simulink model "VisionModel_v16_3"  (Simulink 7.6)
settings: Solver=FixedStepDiscrete  StartTime=0.0  StopTime=0  RelTol=1e-3
undefined symbols (not defined in the file or in its folder): Rec, SDTV
libraries: vipconversions x4, vipgeotforms x3
settings Model: Creator=Administrator  LastModifiedBy=root
settings OptimizationCC: OptimizeModelRefInitCode=on
settings RTWCC: SystemTargetFile=ert.tlc  GenCodeOnly=on  TemplateMakefile=ert_default_tmf  PostCodeGenCommand=packNGo(buildInfo, {'packType' 'flat'})  Description=Real-Time Workshop Embedded Coder  GenerateReport=on  ProcessScript=ert_make_rtw_hook  IncludeHyperlinkInReport=on  LaunchReport=on  TargetLang=C++
settings CodeAppCC: IgnoreCustomStorageClasses=off
settings ERTTargetCC: MultiwordLength=2048  GenerateSampleERTMain=on  IncludeMdlTerminateFcn=off  ERTCustomFileTemplate=example_file_process.tlc  ConvertIfToSwitch=off

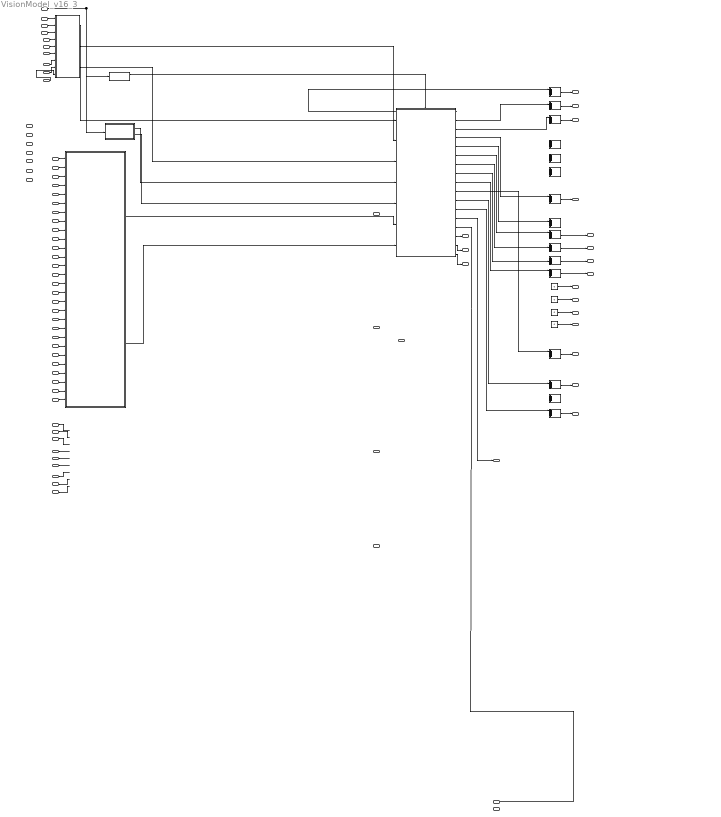
== system VisionModel_v16_3 ==
  note: Forward camera QImage array
  note: Down camera QImage array
  note: Forward
  note: Down
  note: Current target information
  note: Desired target information
  note: Mode and general target information
  note: Note: TargetFound, and the last three inputs to MotionController.mdl,
      | can be changed by the script, not the vision model.
  note: Path-following variables
      | DesiredPathDirection:
      | 0 = Use internal default
      | 1 = Take left path
      | 2 = Take right path
  R_forward_in : Inport  PortDimensions=Forward_Camera_Dimensions
  G_forward_in : Inport  Port=2  PortDimensions=Forward_Camera_Dimensions
  B_forward_in : Inport  Port=3  PortDimensions=Forward_Camera_Dimensions
  R_down_in : Inport  Port=4  PortDimensions=Down_Camera_Dimensions
  G_down_in : Inport  Port=5  PortDimensions=Down_Camera_Dimensions
  B_down_in : Inport  Port=6  PortDimensions=Down_Camera_Dimensions
  ModeSelect : Inport  Port=7
  OutputImage : Inport  Port=8
  DesiredPathDirection : Inport  Port=9
  DesiredBuoyColor : Inport  Port=10
  DesiredTorpedoColor : Inport  Port=11
  white_al : Inport  Port=12
  white_au : Inport  Port=13
  white_bl : Inport  Port=14
  white_bu : Inport  Port=15
  black_al : Inport  Port=16
  black_au : Inport  Port=17
  black_bl : Inport  Port=18
  black_bu : Inport  Port=19
  blue_al : Inport  Port=20
  blue_au : Inport  Port=21
  blue_bl : Inport  Port=22
  blue_bu : Inport  Port=23
  red_al : Inport  Port=24
  red_au : Inport  Port=25
  red_bl : Inport  Port=26
  red_bu : Inport  Port=27
  orange_al : Inport  Port=28
  orange_au : Inport  Port=29
  orange_bl : Inport  Port=30
  orange_bu : Inport  Port=31
  yellow_al : Inport  Port=32
  yellow_au : Inport  Port=33
  yellow_bl : Inport  Port=34
  yellow_bu : Inport  Port=35
  green_al : Inport  Port=36
  green_au : Inport  Port=37
  green_bl : Inport  Port=38
  green_bu : Inport  Port=39
  black_override : Inport  Port=40
  white_override : Inport  Port=41
  blue_override : Inport  Port=42
  red_override : Inport  Port=43
  orange_override : Inport  Port=44
  yellow_override : Inport  Port=45
  green_override : Inport  Port=46
  Scale_Forward_R : Inport  Port=47
  Scale_Forward_G : Inport  Port=48
  Scale_Forward_B : Inport  Port=49
  Scale_Forward_H : Inport  Port=50
  Scale_Forward_S : Inport  Port=51
  Scale_Forward_V : Inport  Port=52
  Scale_Down_R : Inport  Port=53
  Scale_Down_G : Inport  Port=54
  Scale_Down_B : Inport  Port=55
  Scale_Down_H : Inport  Port=56
  Scale_Down_S : Inport  Port=57
  Scale_Down_V : Inport  Port=58
  DeadReckonHeading : Inport  Port=59
  Add{,2..6,18..27} (16 alike) : Sum  Inputs=++++++
  Blob_Analysis : Subsystem  TreatAsAtomicUnit=on
  ColorSelect : Subsystem  TreatAsAtomicUnit=on
  Constant{,1..3} (4 alike) : Constant  Value=0
  Forward Filter : Subsystem
  If1 : If  IfExpression=u1 == 1 | u1 == 3 | u1 == 4 | u1 == 5  ElseIfExpressions=u1 == 2 | u1 == 6  ShowElse=off
  make_color_range : Stateflow chart  TreatAsAtomicUnit=on
  R_forward_out : Outport  OutDataTypeStr=double
  G_forward_out : Outport  Port=2  OutDataTypeStr=double
  B_forward_out : Outport  Port=3  OutDataTypeStr=double
  R_down_out : Outport  Port=4  OutDataTypeStr=double
  G_down_out : Outport  Port=5  OutDataTypeStr=double
  B_down_out : Outport  Port=6  OutDataTypeStr=double
  TargetSelect : Outport  Port=7  OutDataTypeStr=double
  TargetX : Outport  Port=8  OutDataTypeStr=double
  TargetY : Outport  Port=9  OutDataTypeStr=double
  TargetZ : Outport  Port=10  OutDataTypeStr=double
  TargetYaw : Outport  Port=11  OutDataTypeStr=double
  DesiredTargetX : Outport  Port=12  OutDataTypeStr=double
  DesiredTargetY : Outport  Port=13  OutDataTypeStr=double
  DesiredTargetZ : Outport  Port=14  OutDataTypeStr=double
  DesiredTargetYaw : Outport  Port=15  OutDataTypeStr=double
  TargetDetected : Outport  Port=16  OutDataTypeStr=double
  PathState : Outport  Port=17  OutDataTypeStr=double
  BuoyColors : Outport  Port=18  OutDataTypeStr=double
  FireAuthorization : Outport  Port=19  OutDataTypeStr=double
  TargetType : Outport  Port=20  OutDataTypeStr=double
  TargetSize : Outport  Port=21  OutDataTypeStr=double
  wires:
  G_down_in/1 -> ?
  R_down_in/1 -> ?
  B_down_in/1 -> ?
  R_forward_in/1 -> Forward Filter/1(R_in)
  G_forward_in/1 -> Forward Filter/2(G_in)
  B_forward_in/1 -> Forward Filter/3(B_in)
  Add3/1 -> TargetX/1
  Add4/1 -> TargetY/1
  Add5/1 -> TargetZ/1
  Add6/1 -> TargetYaw/1
  Add19/1 -> PathState/1
  Constant/1 -> DesiredTargetX/1
  Constant3/1 -> DesiredTargetYaw/1
  Constant2/1 -> DesiredTargetZ/1
  Constant1/1 -> DesiredTargetY/1
  Add21/1 -> FireAuthorization/1
  ModeSelect/1 -> If1/1, ColorSelect/1(ModeSelect)
  Add/1 -> TargetSelect/1
  Add18/1 -> TargetDetected/1
  white_al/1 -> make_color_range/1(white_al)
  white_au/1 -> make_color_range/2(white_au)
  white_bl/1 -> make_color_range/3(white_bl)
  white_bu/1 -> make_color_range/4(white_bu)
  black_al/1 -> make_color_range/5(black_al)
  black_au/1 -> make_color_range/6(black_au)
  black_bl/1 -> make_color_range/7(black_bl)
  black_bu/1 -> make_color_range/8(black_bu)
  blue_al/1 -> make_color_range/9(blue_al)
  blue_au/1 -> make_color_range/10(blue_au)
  blue_bl/1 -> make_color_range/11(blue_bl)
  blue_bu/1 -> make_color_range/12(blue_bu)
  red_al/1 -> make_color_range/13(red_al)
  red_au/1 -> make_color_range/14(red_au)
  red_bl/1 -> make_color_range/15(red_bl)
  red_bu/1 -> make_color_range/16(red_bu)
  orange_al/1 -> make_color_range/17(orange_al)
  orange_au/1 -> make_color_range/18(orange_au)
  orange_bl/1 -> make_color_range/19(orange_bl)
  orange_bu/1 -> make_color_range/20(orange_bu)
  yellow_al/1 -> make_color_range/21(yellow_al)
  yellow_au/1 -> make_color_range/22(yellow_au)
  yellow_bl/1 -> make_color_range/23(yellow_bl)
  yellow_bu/1 -> make_color_range/24(yellow_bu)
  green_al/1 -> make_color_range/25(green_al)
  green_au/1 -> make_color_range/26(green_au)
  green_bl/1 -> make_color_range/27(green_bl)
  green_bu/1 -> make_color_range/28(green_bu)
  make_color_range/1(a_range) -> Blob_Analysis/6(a_range)
  Forward Filter/1(R_out) -> Blob_Analysis/1(R_in)
  Forward Filter/2(G_out) -> Blob_Analysis/2(G_in)
  Forward Filter/3(B_out) -> Blob_Analysis/3(B_in)
  ColorSelect/1(ColorFilter) -> Blob_Analysis/4(ColorFilter)
  ColorSelect/2(OutputSegmentedImage) -> Blob_Analysis/5(OutputSegmentedImage)
  make_color_range/2(b_range) -> Blob_Analysis/7(b_range)
  If1/1 -> Blob_Analysis/Action
  Add22/1 -> R_forward_out/1
  Add23/1 -> G_forward_out/1
  Add24/1 -> B_forward_out/1
  Scale_Forward_R/1 -> Forward Filter/4(Scale_Forward_R)
  Scale_Forward_G/1 -> Forward Filter/5(Scale_Forward_G)
  Scale_Forward_B/1 -> Forward Filter/6(Scale_Forward_B)
  Scale_Forward_H/1 -> Forward Filter/7(Scale_Forward_H)
  Scale_Forward_S/1 -> Forward Filter/8(Scale_Forward_S)
  Scale_Forward_V/1 -> Forward Filter/9(Scale_Forward_V)
  Scale_Down_R/1 -> ?
  Scale_Down_G/1 -> ?
  Scale_Down_B/1 -> ?
  Scale_Down_H/1 -> ?
  Scale_Down_S/1 -> ?
  Scale_Down_V/1 -> ?
  Blob_Analysis/1(BlobHues) -> Add22/1
  Blob_Analysis/2(Area) -> Add23/2
  Blob_Analysis/3(Centroid) -> Add24/1
  Blob_Analysis/4(BBox) -> Add/1
  Blob_Analysis/5(MajorAxis) -> Add2/2
  Blob_Analysis/6(MinorAxis) -> Add3/1
  Blob_Analysis/7(Orientation) -> Add4/3
  Blob_Analysis/8(Eccentricity) -> Add5/4
  Blob_Analysis/9(Extent) -> Add6/1
  Blob_Analysis/10(BlobCount) -> Add18/1
  Blob_Analysis/11(BlobColor) -> Add19/2
  Blob_Analysis/12(bw_image) -> Add21/1
  Blob_Analysis/13(num_colors) -> BuoyColors/1
  Blob_Analysis/14(ref_colors) -> TargetType/1
  Blob_Analysis/15(R_out) -> R_down_out/1
  Blob_Analysis/16(G_out) -> G_down_out/1
  Blob_Analysis/17(B_out) -> B_down_out/1

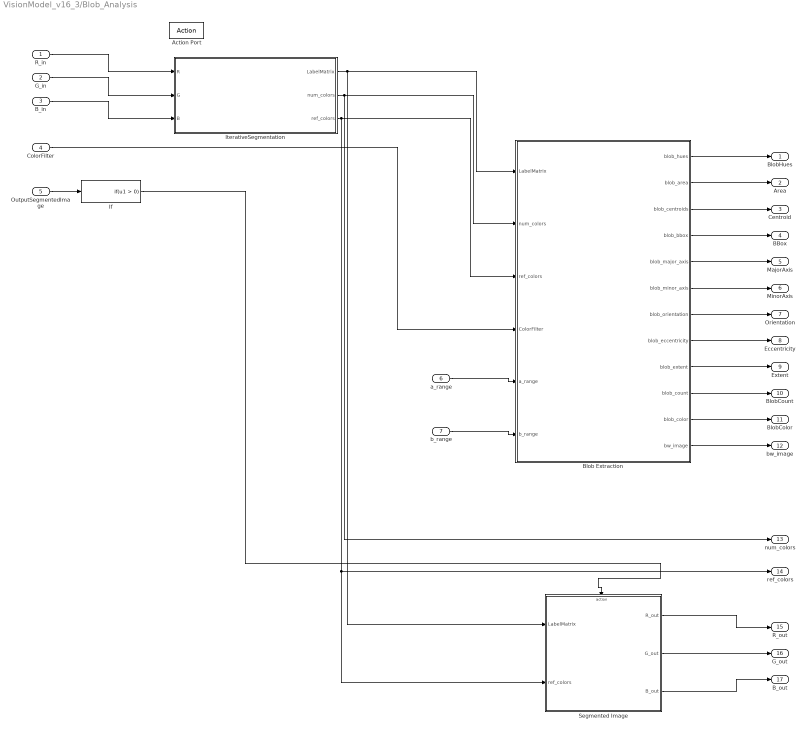
== system VisionModel_v16_3/Blob_Analysis ==
  R_in : Inport
  G_in : Inport  Port=2
  B_in : Inport  Port=3
  ColorFilter : Inport  Port=4
  OutputSegmentedImage : Inport  Port=5
  a_range : Inport  Port=6
  b_range : Inport  Port=7
  Action Port : ActionPort  ActionType=then
  Blob Extraction : Stateflow chart  TreatAsAtomicUnit=on
  If : If  ShowElse=off
  IterativeSegmentation : Subsystem
      settings: UndoDeleteFcn=Stateflow.SLINSF.SimulinkMan.restorePreDeleteFcn  PreDeleteFcn=Stateflow.SLINSF.SimulinkMan.removePreDeleteFcn
  Segmented Image : Subsystem  TreatAsAtomicUnit=on
  BlobHues : Outport
  Area : Outport  Port=2
  Centroid : Outport  Port=3
  BBox : Outport  Port=4
  MajorAxis : Outport  Port=5
  MinorAxis : Outport  Port=6
  Orientation : Outport  Port=7
  Eccentricity : Outport  Port=8
  Extent : Outport  Port=9
  BlobCount : Outport  Port=10
  BlobColor : Outport  Port=11
  bw_image : Outport  Port=12
  num_colors : Outport  Port=13
  ref_colors : Outport  Port=14
  R_out : Outport  Port=15
  G_out : Outport  Port=16
  B_out : Outport  Port=17
  wires:
  Blob Extraction/12(bw_image) -> bw_image/1
  Blob Extraction/10(blob_count) -> BlobCount/1
  Blob Extraction/9(blob_extent) -> Extent/1
  Blob Extraction/8(blob_eccentricity) -> Eccentricity/1
  Blob Extraction/7(blob_orientation) -> Orientation/1
  Blob Extraction/6(blob_minor_axis) -> MinorAxis/1
  Blob Extraction/5(blob_major_axis) -> MajorAxis/1
  Blob Extraction/4(blob_bbox) -> BBox/1
  Blob Extraction/3(blob_centroids) -> Centroid/1
  Blob Extraction/2(blob_area) -> Area/1
  Blob Extraction/1(blob_hues) -> BlobHues/1
  ColorFilter/1 -> Blob Extraction/4(ColorFilter)
  a_range/1 -> Blob Extraction/5(a_range)
  b_range/1 -> Blob Extraction/6(b_range)
  IterativeSegmentation/1(LabelMatrix) -> Blob Extraction/1(LabelMatrix), Segmented Image/1(LabelMatrix)
  IterativeSegmentation/2(num_colors) -> Blob Extraction/2(num_colors), num_colors/1
  IterativeSegmentation/3(ref_colors) -> Blob Extraction/3(ref_colors), Segmented Image/2(ref_colors), ref_colors/1
  R_in/1 -> IterativeSegmentation/1(R)
  G_in/1 -> IterativeSegmentation/2(G)
  B_in/1 -> IterativeSegmentation/3(B)
  If/1 -> Segmented Image/Action
  OutputSegmentedImage/1 -> If/1
  Segmented Image/1(R_out) -> R_out/1
  Segmented Image/2(G_out) -> G_out/1
  Segmented Image/3(B_out) -> B_out/1
  Blob Extraction/11(blob_color) -> BlobColor/1

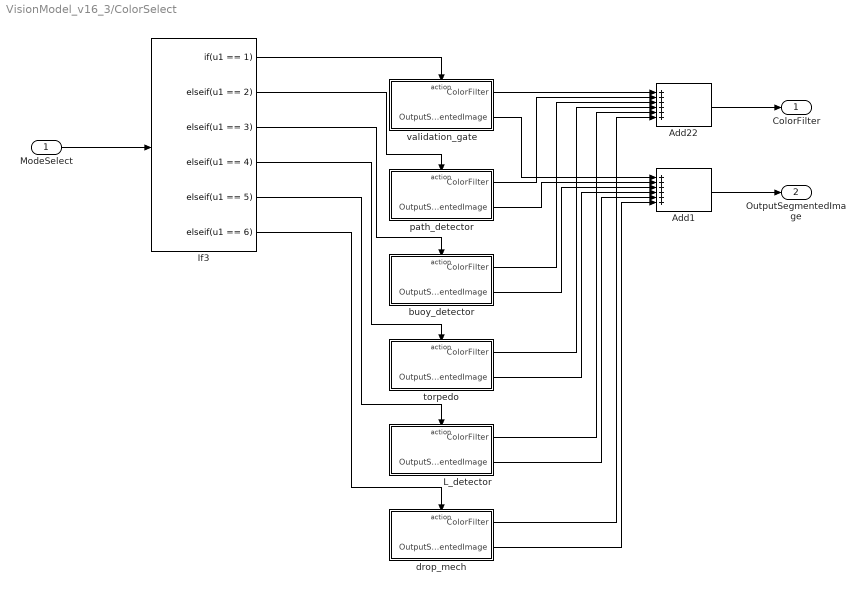
== system VisionModel_v16_3/ColorSelect ==
  ModeSelect : Inport
  Add1 : Sum  Inputs=++++++
  Add22 : Sum  Inputs=++++++
  If3 : If  IfExpression=u1 == 1  ElseIfExpressions=u1 == 2, u1 == 3, u1 == 4, u1 == 5, u1 == 6  ShowElse=off
  L_detector : Subsystem  TreatAsAtomicUnit=on
  buoy_detector : Subsystem  TreatAsAtomicUnit=on
  drop_mech : Subsystem  TreatAsAtomicUnit=on
  path_detector : Subsystem  TreatAsAtomicUnit=on
  torpedo : Subsystem  TreatAsAtomicUnit=on
  validation_gate : Subsystem  TreatAsAtomicUnit=on
  ColorFilter : Outport  OutDataTypeStr=double
  OutputSegmentedImage : Outport  Port=2  OutDataTypeStr=double
  wires:
  ModeSelect/1 -> If3/1
  If3/1 -> validation_gate/Action
  Add22/1 -> ColorFilter/1
  If3/2 -> path_detector/Action
  If3/3 -> buoy_detector/Action
  If3/4 -> torpedo/Action
  If3/5 -> L_detector/Action
  If3/6 -> drop_mech/Action
  Add1/1 -> OutputSegmentedImage/1
  validation_gate/1(ColorFilter) -> Add22/1
  validation_gate/2(OutputSegmentedImage) -> Add1/1
  path_detector/1(ColorFilter) -> Add22/2
  path_detector/2(OutputSegmentedImage) -> Add1/2
  buoy_detector/1(ColorFilter) -> Add22/3
  buoy_detector/2(OutputSegmentedImage) -> Add1/3
  torpedo/1(ColorFilter) -> Add22/4
  torpedo/2(OutputSegmentedImage) -> Add1/4
  L_detector/1(ColorFilter) -> Add22/5
  L_detector/2(OutputSegmentedImage) -> Add1/5
  drop_mech/1(ColorFilter) -> Add22/6
  drop_mech/2(OutputSegmentedImage) -> Add1/6

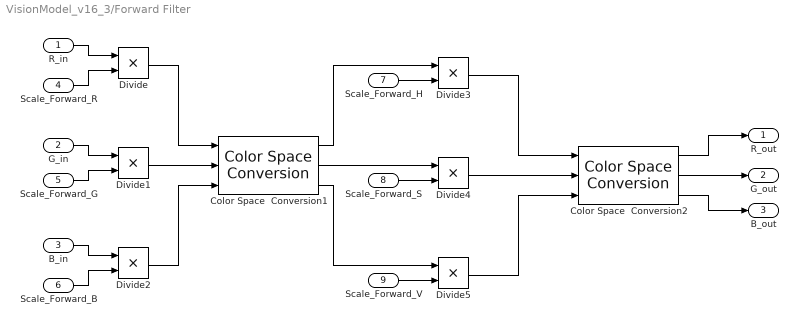
== system VisionModel_v16_3/Forward Filter ==
  R_in : Inport  PortDimensions=Forward_Camera_Dimensions
  G_in : Inport  Port=2  PortDimensions=Forward_Camera_Dimensions
  B_in : Inport  Port=3  PortDimensions=Forward_Camera_Dimensions
  Scale_Forward_R : Inport  Port=4
  Scale_Forward_G : Inport  Port=5
  Scale_Forward_B : Inport  Port=6
  Scale_Forward_H : Inport  Port=7
  Scale_Forward_S : Inport  Port=8
  Scale_Forward_V : Inport  Port=9
  Color Space  Conversion1 : vipconversions/Color Space  Conversion  conversion=Obsolete  conversionActive=R'G'B' to HSV  wp_str=D50  rec=Rec. 601 (SDTV)  sys=1125/60/2:1  imagePorts=Separate color signals
  Color Space  Conversion2 : vipconversions/Color Space  Conversion  conversion=Obsolete  conversionActive=HSV to R'G'B'  wp_str=D50  rec=Rec. 601 (SDTV)  sys=1125/60/2:1  imagePorts=Separate color signals
  Divide{,1..5} (6 alike) : Product  Inputs=**
  R_out : Outport  OutDataTypeStr=double
  G_out : Outport  Port=2  OutDataTypeStr=double
  B_out : Outport  Port=3  OutDataTypeStr=double
  wires:
  Color Space  Conversion2/1 -> R_out/1
  Color Space  Conversion2/2 -> G_out/1
  Color Space  Conversion2/3 -> B_out/1
  R_in/1 -> Divide/1
  Scale_Forward_R/1 -> Divide/2
  G_in/1 -> Divide1/1
  Scale_Forward_G/1 -> Divide1/2
  B_in/1 -> Divide2/1
  Scale_Forward_B/1 -> Divide2/2
  Divide/1 -> Color Space  Conversion1/1
  Divide1/1 -> Color Space  Conversion1/2
  Divide2/1 -> Color Space  Conversion1/3
  Scale_Forward_H/1 -> Divide3/2
  Scale_Forward_S/1 -> Divide4/2
  Scale_Forward_V/1 -> Divide5/2
  Color Space  Conversion1/1 -> Divide3/1
  Color Space  Conversion1/2 -> Divide4/1
  Color Space  Conversion1/3 -> Divide5/1
  Divide4/1 -> Color Space  Conversion2/2
  Divide3/1 -> Color Space  Conversion2/1
  Divide5/1 -> Color Space  Conversion2/3

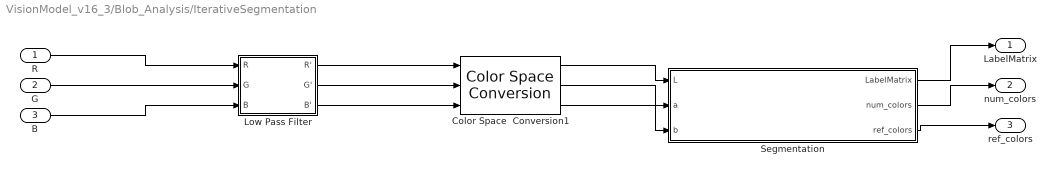
== system VisionModel_v16_3/Blob_Analysis/IterativeSegmentation ==
  R : Inport
  G : Inport  Port=2
  B : Inport  Port=3
  Color Space  Conversion1 : vipconversions/Color Space  Conversion  conversion=Obsolete  conversionActive=sR'G'B' to L*a*b*  wp_str=D50  rec=Rec. 601 (SDTV)  sys=1125/60/2:1  imagePorts=Separate color signals
  Low Pass Filter : Subsystem
  Segmentation : Subsystem
  LabelMatrix : Outport
  num_colors : Outport  Port=2
  ref_colors : Outport  Port=3
  wires:
  Low Pass Filter/3(B') -> Color Space  Conversion1/3
  Low Pass Filter/2(G') -> Color Space  Conversion1/2
  Low Pass Filter/1(R') -> Color Space  Conversion1/1
  Color Space  Conversion1/3 -> Segmentation/3(b)
  Color Space  Conversion1/2 -> Segmentation/2(a)
  Color Space  Conversion1/1 -> Segmentation/1(L)
  R/1 -> Low Pass Filter/1(R)
  G/1 -> Low Pass Filter/2(G)
  B/1 -> Low Pass Filter/3(B)
  Segmentation/1(LabelMatrix) -> LabelMatrix/1
  Segmentation/2(num_colors) -> num_colors/1
  Segmentation/3(ref_colors) -> ref_colors/1

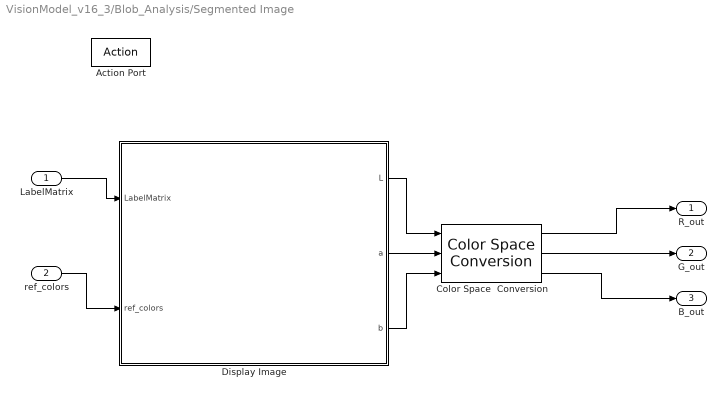
== system VisionModel_v16_3/Blob_Analysis/Segmented Image ==
  LabelMatrix : Inport
  ref_colors : Inport  Port=2
  Action Port : ActionPort  ActionType=then
  Color Space  Conversion : vipconversions/Color Space  Conversion  conversion=Obsolete  conversionActive=L*a*b* to sR'G'B'  wp_str=D65  rec=Rec. 601 (SDTV)  sys=1125/60/2:1  imagePorts=Separate color signals
  Display Image : Stateflow chart  TreatAsAtomicUnit=on
  R_out : Outport
  G_out : Outport  Port=2
  B_out : Outport  Port=3
  wires:
  LabelMatrix/1 -> Display Image/1(LabelMatrix)
  ref_colors/1 -> Display Image/2(ref_colors)
  Display Image/1(L) -> Color Space  Conversion/1
  Display Image/2(a) -> Color Space  Conversion/2
  Display Image/3(b) -> Color Space  Conversion/3
  Color Space  Conversion/1 -> R_out/1
  Color Space  Conversion/2 -> G_out/1
  Color Space  Conversion/3 -> B_out/1

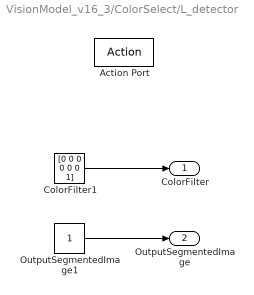
== system VisionModel_v16_3/ColorSelect/L_detector ==
  Action Port : ActionPort  ActionType=elseif
  ColorFilter1 : Constant  Value=[0 0 0 0 0 0 1]  SampleTime=-1
  OutputSegmentedImage1 : Constant  SampleTime=-1
  ColorFilter : Outport  OutDataTypeStr=double
  OutputSegmentedImage : Outport  Port=2  OutDataTypeStr=double
  wires:
  ColorFilter1/1 -> ColorFilter/1
  OutputSegmentedImage1/1 -> OutputSegmentedImage/1

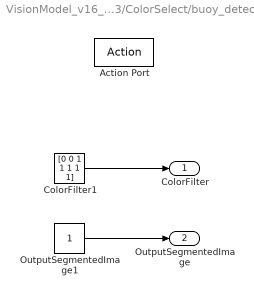
== system VisionModel_v16_3/ColorSelect/buoy_detector ==
  Action Port : ActionPort  ActionType=elseif
  ColorFilter1 : Constant  Value=[0 0 1 1 1 1 1]  SampleTime=-1
  OutputSegmentedImage1 : Constant  SampleTime=-1
  ColorFilter : Outport  OutDataTypeStr=double
  OutputSegmentedImage : Outport  Port=2  OutDataTypeStr=double
  wires:
  ColorFilter1/1 -> ColorFilter/1
  OutputSegmentedImage1/1 -> OutputSegmentedImage/1

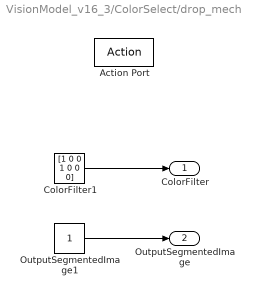
== system VisionModel_v16_3/ColorSelect/drop_mech ==
  Action Port : ActionPort  ActionType=elseif
  ColorFilter1 : Constant  Value=[1 0 0 1 0 0 0]  SampleTime=-1
  OutputSegmentedImage1 : Constant  SampleTime=-1
  ColorFilter : Outport  OutDataTypeStr=double
  OutputSegmentedImage : Outport  Port=2  OutDataTypeStr=double
  wires:
  OutputSegmentedImage1/1 -> OutputSegmentedImage/1
  ColorFilter1/1 -> ColorFilter/1

== system VisionModel_v16_3/ColorSelect/path_detector ==
  Action Port : ActionPort  ActionType=elseif
  ColorFilter1 : Constant  Value=[0 0 0 1 1 1 0]  SampleTime=-1
  OutputSegmentedImage1 : Constant  SampleTime=-1
  ColorFilter : Outport  OutDataTypeStr=double
  OutputSegmentedImage : Outport  Port=2  OutDataTypeStr=double
  wires:
  OutputSegmentedImage1/1 -> OutputSegmentedImage/1
  ColorFilter1/1 -> ColorFilter/1

== system VisionModel_v16_3/ColorSelect/torpedo ==
  Action Port : ActionPort  ActionType=elseif
  ColorFilter1 : Constant  Value=[0 0 1 1 0 0 0]  SampleTime=-1
  OutputSegmentedImage1 : Constant  SampleTime=-1
  ColorFilter : Outport  OutDataTypeStr=double
  OutputSegmentedImage : Outport  Port=2  OutDataTypeStr=double
  wires:
  OutputSegmentedImage1/1 -> OutputSegmentedImage/1
  ColorFilter1/1 -> ColorFilter/1

== system VisionModel_v16_3/ColorSelect/validation_gate ==
  Action Port : ActionPort  ActionType=then
  ColorFilter1 : Constant  Value=[0 1 0 0 1 0 0]  SampleTime=-1
  OutputSegmentedImage1 : Constant  SampleTime=-1
  ColorFilter : Outport  OutDataTypeStr=double
  OutputSegmentedImage : Outport  Port=2  OutDataTypeStr=double
  wires:
  ColorFilter1/1 -> ColorFilter/1
  OutputSegmentedImage1/1 -> OutputSegmentedImage/1

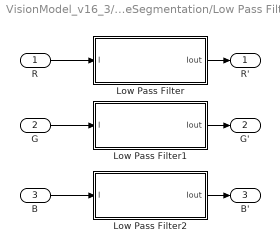
== system VisionModel_v16_3/Blob_Analysis/IterativeSegmentation/Low Pass Filter ==
  R : Inport
  G : Inport  Port=2
  B : Inport  Port=3
  Low Pass Filter : Stateflow chart  TreatAsAtomicUnit=on
  Low Pass Filter1 : Stateflow chart  TreatAsAtomicUnit=on
  Low Pass Filter2 : Stateflow chart  TreatAsAtomicUnit=on
  R' : Outport
  G' : Outport  Port=2
  B' : Outport  Port=3
  wires:
  Low Pass Filter/1(Iout) -> R'/1
  Low Pass Filter2/1(Iout) -> B'/1
  Low Pass Filter1/1(Iout) -> G'/1
  B/1 -> Low Pass Filter2/1(I)
  G/1 -> Low Pass Filter1/1(I)
  R/1 -> Low Pass Filter/1(I)

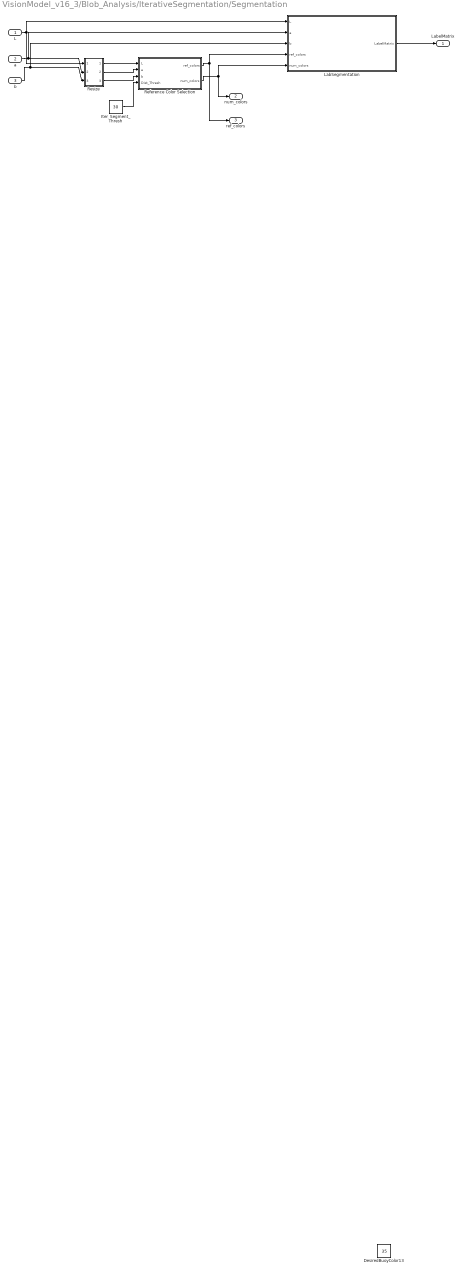
== system VisionModel_v16_3/Blob_Analysis/IterativeSegmentation/Segmentation ==
  L : Inport
  a : Inport  Port=2
  b : Inport  Port=3
  DesiredBuoyColor13 : Constant  Value=35  SampleTime=-1
  Iter_Segment_Thresh : Constant  Value=30  SampleTime=-1
  LabSegmentation : Stateflow chart  TreatAsAtomicUnit=on
  Reference Color Selection : Stateflow chart  TreatAsAtomicUnit=on
  Resize : Subsystem
  LabelMatrix : Outport
  num_colors : Outport  Port=2
  ref_colors : Outport  Port=3
  wires:
  LabSegmentation/1(LabelMatrix) -> LabelMatrix/1
  Reference Color Selection/2(num_colors) -> LabSegmentation/5(num_colors), num_colors/1
  Reference Color Selection/1(ref_colors) -> ref_colors/1, LabSegmentation/4(ref_colors)
  Resize/3(Out3) -> Reference Color Selection/3(b)
  Resize/2(Out2) -> Reference Color Selection/2(a)
  Resize/1(Out1) -> Reference Color Selection/1(L)
  b/1 -> LabSegmentation/3(b), Resize/3(In3)
  a/1 -> LabSegmentation/2(a), Resize/2(In2)
  L/1 -> LabSegmentation/1(L), Resize/1(In1)
  Iter_Segment_Thresh/1 -> Reference Color Selection/4(Dist_Thresh)

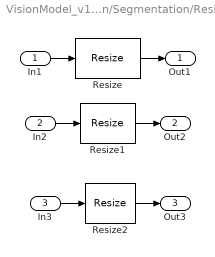
== system VisionModel_v16_3/Blob_Analysis/IterativeSegmentation/Segmentation/Resize ==
  In1 : Inport
  In2 : Inport  Port=2
  In3 : Inport  Port=3
  Resize : vipgeotforms/Resize  DialogController=vipDDGCreate  DialogControllerArgs=DataTag0  specify=Number of output rows and columns  rfactor=[]  outCols=25  outRows=25  outRowsCols=[60 80]  interp_method=Bilinear  antialias=on  useROI=off  roiFlag=off  prodOutputMode=Binary point scaling  prodOutputWordLength=32  prodOutputFracLength=10  roundingMode=Nearest  overflowMode=on
  Resize1 : vipgeotforms/Resize  DialogController=vipDDGCreate  DialogControllerArgs=DataTag1  specify=Number of output rows and columns  rfactor=[200 150]  outCols=25  outRows=25  outRowsCols=[60 80]  interp_method=Bilinear  antialias=on  useROI=off  roiFlag=off  prodOutputMode=Binary point scaling  prodOutputWordLength=32  prodOutputFracLength=10  roundingMode=Nearest  overflowMode=on
  Resize2 : vipgeotforms/Resize  DialogController=vipDDGCreate  DialogControllerArgs=DataTag2  specify=Number of output rows and columns  rfactor=[200 150]  outCols=25  outRows=25  outRowsCols=[60 80]  interp_method=Bilinear  antialias=on  useROI=off  roiFlag=off  prodOutputMode=Binary point scaling  prodOutputWordLength=32  prodOutputFracLength=10  roundingMode=Nearest  overflowMode=on
  Out1 : Outport
  Out2 : Outport  Port=2
  Out3 : Outport  Port=3
  wires:
  Resize2/1 -> Out3/1
  In3/1 -> Resize2/1
  Resize1/1 -> Out2/1
  In2/1 -> Resize1/1
  Resize/1 -> Out1/1
  In1/1 -> Resize/1

== matlab function Blob_Analysis/Blob Extraction ==
  data: LabelMatrix input double; num_colors input double; ref_colors input double; ColorFilter input double; a_range input double; b_range input double; blob_hues output double; blob_area output double; blob_centroids output double; blob_bbox output double; blob_major_axis output double; blob_minor_axis output double; blob_orientation output double; blob_eccentricity output double; blob_extent output double; blob_count output double; blob_color output double; bw_image output double
function [blob_hues, blob_area, blob_centroids, blob_bbox, blob_major_axis, blob_minor_axis, blob_orientation, blob_eccentricity, blob_extent, blob_count, blob_color, bw_image] = GetBlobInfo(LabelMatrix, num_colors, ref_colors, ColorFilter, a_range, b_range)
% This function calculates blob information for each color component after
%   iterative segmentation


% Output
%   blob_color = 1xN vector of color indices (global color scheme)


% Initialize
max_num_blobs = 50;
min_blob_area = 5;

[rows, cols] = size(LabelMatrix);
image_area = rows*cols;
LogicMatrix = false(rows,cols);
bw_image = zeros(rows,cols);

blob_hues = zeros(3,max_num_blobs);
blob_area = -1.*ones(1,max_num_blobs);
blob_bbox = zeros(4,max_num_blobs);
blob_major_axis = zeros(1,max_num_blobs);
blob_minor_axis = zeros(1,max_num_blobs);
blob_centroids = zeros(2,max_num_blobs);
blob_eccentricity = zeros(1,max_num_blobs);
blob_extent = zeros(1,max_num_blobs);
blob_orientation = zeros(1,max_num_blobs);
blob_count = 0;

blob_color = zeros(1,max_num_blobs);

max_num_col_filter = length(ColorFilter);
num_col_filter = sum(ColorFilter);

area_thresh = .1;


% Determine L_white and L_black as needed
find_white = 0;
find_black = 0;
L_white = 101;
L_black = -1;
color_areas = zeros(1,size(ref_colors,1));

if(ColorFilter(1) + ColorFilter(2) > 0)
    for row = 1:rows
        for col = 1:cols
            color_areas(LabelMatrix(row,col)) = color_areas(LabelMatrix(row,col)) + 1;
        end
    end
end

if(ColorFilter(1) == 1)
    
    % Determine the brightest colors, but allow a maximum area
    %   ratio of the image to be "white"
    find_white = 1;
    
    positive_area = 0;
    for n = 1:num_colors
        
        maxL = -1;
        k_max = -1;
        for k = 1:num_colors
            L = ref_colors(k,1);
            if(L > maxL && L < L_white)
                maxL = L;
                k_max = k;
            end
        end
        
        positive_area = positive_area + color_areas(k_max);
        if(positive_area/image_area >= area_thresh && n > 1)
            break;
        end
        
        L_white = maxL;
        
    end
end

if(ColorFilter(2) == 1)
    
    % Determine the darkest colors, but allow a maximum area
    %   ratio of the image to be "black"
    find_black = 1;
    
    for row = 1:rows
        for col = 1:cols
            color_areas(LabelMatrix(row,col)) = color_areas(LabelMatrix(row,col)) + 1;
        end
    end
    
    positive_area = 0;
    for n = 1:num_colors
        
        minL = 101;
        k_min = -1;
        for k = 1:num_colors
            L = ref_colors(k,1);
            if(L < minL && L > L_black)
                minL = L;
                k_min = k;
            end
        end
        
        positive_area = positive_area + color_areas(k_min);
        if(positive_area/image_area >= area_thresh && n > 1)
            break;
        end
        
        L_black = minL;
        
    end
end


% Input hblob, a matrix containing [Area, blob_centroids, Eccentricity] for each
% identified blob
persistent hblob
if isempty(hblob)
    hblob = video.BlobAnalysis('AreaOutputPort',true,'CentroidOutputPort',true,...
        'BoundingBoxOutputPort',true,'MajorAxisLengthOutputPort',true,'MinorAxisLengthOutputPort',true,...
        'OrientationOutputPort',true,...
        'EccentricityOutputPort',true,'ExtentOutputPort',true,'NumBlobsOutputPort',true,...
        'MinimumBlobAreaSource','Property','MinimumBlobArea', min_blob_area);
end


% Calculate geometric information about the blobs
%
% LogicMatrix is a binary version of LabelMatrix, with ones at all
%   locations for which color values are k, and zeros everywhere else
%
% Explanation
%   condition1 == 1 causes the k'th color to be analyzed by blob analysis,
%     as well as be included in the black-and-white image
%   condition1 == 0 disallows both of these items and simply ignores color
%     k
%   condition0 == 1 ensures that condition1 is true for all k
%   condition0 == 0 enforces a filter which allows only the colors
%     specified in the ColorFilter vector
condition0 = (num_col_filter == 0);
current_color = 0;
for k = 1:num_colors
    
    % Decide whether or not to perform blob analysis
    condition1 = 0;
    if(condition0)
        condition1 = 1;
    else
        a = ref_colors(k, 2);
        b = ref_colors(k, 3);
        for i = 1:max_num_col_filter
            
            % Skip colors that have not been specified
            if(ColorFilter(i) == 0)
                continue;
            end
            
            if( find_white == 1 && ref_colors(k,1) >= L_white)  % Handle "white" differently than other colors
                condition1 = 1;
                current_color = 1;
                break;
            elseif( find_black == 1 && ref_colors(k,1) <= L_black)  % Handle "black" differently than other colors
                condition1 = 1;
                current_color = 2;
                break;
            elseif( a >= a_range(1,i) && a <= a_range(2,i) && b >= b_range(1,i) && b <= b_range(2,i) )
                condition1 = 1;
                current_color = i;
                break;
            end
            
        end
    end
    
    % Blob analysis
    if( condition1 == 1 )
        
        for i = 1:rows
            for j = 1:cols
                if(LabelMatrix(i,j) ~= k)
                    LogicMatrix(i,j) = false;
                else
                    LogicMatrix(i,j) = true;
                    bw_image(i,j) = 1;
                end
            end
        end

        [TArea,TCentroid,TBBox,TMajorAxis,TMinorAxis,TOrientation,TEccent,TExtent,TNumBlobs] = step(hblob,LogicMatrix);

        for i = 1:TNumBlobs
            if(blob_count + TNumBlobs <= max_num_blobs)

                blob_centroids(1,blob_count+i) = TCentroid(1,i);
                blob_centroids(2,blob_count+i) = TCentroid(2,i);

                ii = round(blob_centroids(1,blob_count+i));
                jj = round(blob_centroids(2,blob_count+i));

                blob_hues(1,blob_count+i) = ref_colors( LabelMatrix(ii,jj), 1 );
                blob_hues(2,blob_count+i) = ref_colors( LabelMatrix(ii,jj), 2 );
                blob_hues(3,blob_count+i) = ref_colors( LabelMatrix(ii,jj), 3 );

                blob_area(blob_count+i) = TArea(i);
                blob_bbox(blob_count+i) = TBBox(i);
                blob_major_axis(blob_count+i) = TMajorAxis(i);
                blob_minor_axis(blob_count+i) = TMinorAxis(i);
                blob_eccentricity(blob_count+i) = TEccent(i);
                blob_extent(blob_count+i) = TExtent(i);
                blob_orientation(blob_count+i) = TOrientation(i);
                
                blob_color(blob_count+i) = current_color;

            end
        end

        blob_count = blob_count + double(TNumBlobs);

    end
    
end


return

== matlab function Blob_Analysis/IterativeSegmentation/Low Pass Filter/Low Pass Filter ==
  data: I input double; Iout output double
function Iout = GaussianBlurr(I)
% This function calculates the gaussian blur of an intensity image

sigma = sqrt(2);

Grows = 3;    % Gaussian matrix rows
Gcols = 3;    % Gaussian matrix columns

[Irows Icols] = size(I);

Iout = double(zeros(Irows,Icols));

Trows = Irows - Grows + 1;
Tcols = Icols - Gcols + 1;
Itemp = double(zeros(Trows,Tcols));

G = zeros(Grows,Gcols);

FirstRow = ceil(-Grows/2);
LastRow = floor(Grows/2);
FirstCol = ceil(-Gcols/2);
LastCol = floor(Gcols/2);
Gsum = 0;
for i=FirstRow:LastRow
    for j = FirstCol:LastCol
        G(i-FirstRow+1,j-FirstCol+1) = exp(-(j*j+i*i)/(2*sigma*sigma));
        Gsum = Gsum + G(i-FirstRow+1,j-FirstCol+1);
    end
end

G = G./Gsum;

Itemp = conv2(double(I),double(G),'valid');

% reflect boundaries to keep image the same size
% top
Iout((1:LastRow),(LastCol+1:Icols-LastCol)) = Itemp((1:LastRow),(1:Tcols));
% bottom
Iout((Irows-LastRow+1:Irows),(LastCol+1:Icols-LastCol)) = Itemp((Trows-LastRow+1:Trows),(1:Tcols));
% left
Iout((1+LastRow:Irows-LastRow),(1:LastCol)) = Itemp((1:Trows),(1:LastCol));
% right
Iout((1+LastRow:Irows-LastRow),(Icols-LastCol+1:Icols)) = Itemp((1:Trows),(Tcols-LastCol+1:Tcols));
% center
Iout((1+LastRow:Irows-LastRow),(1+LastCol:Icols-LastCol)) = Itemp;
% top left corner
Iout(1:LastRow,1:LastCol) = Itemp(1:LastRow,1:LastCol);
% top right corner
Iout(1:LastRow,Icols-LastCol:Icols) = Itemp(1:LastRow,Tcols-LastCol:Tcols);
% bottom left corner
Iout(Irows-LastRow:Irows,1:LastCol) = Itemp(Trows-LastRow:Trows,1:LastCol);
% bottom right corner
Iout(Irows-LastRow:Irows,Icols-LastCol:Icols) = Itemp(Trows-LastRow:Trows,Tcols-LastCol:Tcols);

return

== matlab function Blob_Analysis/IterativeSegmentation/Low Pass Filter/Low Pass Filter1 ==
  data: I input double; Iout output double
function Iout = GaussianBlurr(I)
% This function calculates the gaussian blur of an intensity image

sigma = sqrt(2);

Grows = 3;    % Gaussian matrix rows
Gcols = 3;    % Gaussian matrix columns

[Irows Icols] = size(I);

Iout = double(zeros(Irows,Icols));

Trows = Irows - Grows + 1;
Tcols = Icols - Gcols + 1;
Itemp = double(zeros(Trows,Tcols));

G = zeros(Grows,Gcols);

FirstRow = ceil(-Grows/2);
LastRow = floor(Grows/2);
FirstCol = ceil(-Gcols/2);
LastCol = floor(Gcols/2);
Gsum = 0;
for i=FirstRow:LastRow
    for j = FirstCol:LastCol
        G(i-FirstRow+1,j-FirstCol+1) = exp(-(j*j+i*i)/(2*sigma*sigma));
        Gsum = Gsum + G(i-FirstRow+1,j-FirstCol+1);
    end
end

G = G./Gsum;

Itemp = conv2(double(I),double(G),'valid');

% reflect boundaries to keep image the same size
% top
Iout((1:LastRow),(LastCol+1:Icols-LastCol)) = Itemp((1:LastRow),(1:Tcols));
% bottom
Iout((Irows-LastRow+1:Irows),(LastCol+1:Icols-LastCol)) = Itemp((Trows-LastRow+1:Trows),(1:Tcols));
% left
Iout((1+LastRow:Irows-LastRow),(1:LastCol)) = Itemp((1:Trows),(1:LastCol));
% right
Iout((1+LastRow:Irows-LastRow),(Icols-LastCol+1:Icols)) = Itemp((1:Trows),(Tcols-LastCol+1:Tcols));
% center
Iout((1+LastRow:Irows-LastRow),(1+LastCol:Icols-LastCol)) = Itemp;
% top left corner
Iout(1:LastRow,1:LastCol) = Itemp(1:LastRow,1:LastCol);
% top right corner
Iout(1:LastRow,Icols-LastCol:Icols) = Itemp(1:LastRow,Tcols-LastCol:Tcols);
% bottom left corner
Iout(Irows-LastRow:Irows,1:LastCol) = Itemp(Trows-LastRow:Trows,1:LastCol);
% bottom right corner
Iout(Irows-LastRow:Irows,Icols-LastCol:Icols) = Itemp(Trows-LastRow:Trows,Tcols-LastCol:Tcols);

return

== matlab function Blob_Analysis/IterativeSegmentation/Low Pass Filter/Low Pass Filter2 ==
  data: I input double; Iout output double
function Iout = GaussianBlurr(I)
% This function calculates the gaussian blur of an intensity image

sigma = sqrt(2);

Grows = 3;    % Gaussian matrix rows
Gcols = 3;    % Gaussian matrix columns

[Irows Icols] = size(I);

Iout = double(zeros(Irows,Icols));

Trows = Irows - Grows + 1;
Tcols = Icols - Gcols + 1;
Itemp = double(zeros(Trows,Tcols));

G = zeros(Grows,Gcols);

FirstRow = ceil(-Grows/2);
LastRow = floor(Grows/2);
FirstCol = ceil(-Gcols/2);
LastCol = floor(Gcols/2);
Gsum = 0;
for i=FirstRow:LastRow
    for j = FirstCol:LastCol
        G(i-FirstRow+1,j-FirstCol+1) = exp(-(j*j+i*i)/(2*sigma*sigma));
        Gsum = Gsum + G(i-FirstRow+1,j-FirstCol+1);
    end
end

G = G./Gsum;

Itemp = conv2(double(I),double(G),'valid');

% reflect boundaries to keep image the same size
% top
Iout((1:LastRow),(LastCol+1:Icols-LastCol)) = Itemp((1:LastRow),(1:Tcols));
% bottom
Iout((Irows-LastRow+1:Irows),(LastCol+1:Icols-LastCol)) = Itemp((Trows-LastRow+1:Trows),(1:Tcols));
% left
Iout((1+LastRow:Irows-LastRow),(1:LastCol)) = Itemp((1:Trows),(1:LastCol));
% right
Iout((1+LastRow:Irows-LastRow),(Icols-LastCol+1:Icols)) = Itemp((1:Trows),(Tcols-LastCol+1:Tcols));
% center
Iout((1+LastRow:Irows-LastRow),(1+LastCol:Icols-LastCol)) = Itemp;
% top left corner
Iout(1:LastRow,1:LastCol) = Itemp(1:LastRow,1:LastCol);
% top right corner
Iout(1:LastRow,Icols-LastCol:Icols) = Itemp(1:LastRow,Tcols-LastCol:Tcols);
% bottom left corner
Iout(Irows-LastRow:Irows,1:LastCol) = Itemp(Trows-LastRow:Trows,1:LastCol);
% bottom right corner
Iout(Irows-LastRow:Irows,Icols-LastCol:Icols) = Itemp(Trows-LastRow:Trows,Tcols-LastCol:Tcols);

return

== matlab function Blob_Analysis/IterativeSegmentation/Segmentation/LabSegmentation ==
  data: L input double; LabelMatrix output double; a input double; b input double; ref_colors input double; num_colors input double
function LabelMatrix  = LabSegmentation(L,a,b,ref_colors,num_colors)
% This function generates the label matrix

[rows cols] = size(L);
LabelMatrix = zeros(rows,cols);

for i = 1:rows
    for j = 1:cols
        min_dist = 1000;
        index = 1;
        for k = 1:num_colors
            dist = sqrt((ref_colors(k,1) - L(i,j))^2 + (ref_colors(k,2) - a(i,j))^2 + (ref_colors(k,3) - b(i,j))^2);
            if(dist < min_dist)
                min_dist = double(dist);
                index = k;
            end
        end
        LabelMatrix(i,j) = index;
    end
end


return

== matlab function Blob_Analysis/IterativeSegmentation/Segmentation/Reference Color Selection ==
  data: L input double; ref_colors output double; a input double; b input double; num_colors output double; Dist_Thresh input double
function [ref_colors, num_colors] = Segmentation(L,a,b,Dist_Thresh)
% This function tries segmentation by adding new reference colors everytime
% a pixel is found with a distance greater than a certain amount from
% every other reference color

[rows cols] = size(L);

Dist_Threshold = Dist_Thresh;% L = 0 to 100, a = -100 to 100, b = -100 to 100
                    % max dist = 300 -> 60/300 is 20%
x = 1;  % coefficients determining distance calculation
y = 1.5;
z = 1.5;

max_num_colors = 50;
ref_colors = zeros(max_num_colors,3);   % At most 50 different reference colors
LabelMatrix = zeros(rows,cols);
num_colors = 1;

center_row = floor(rows/2);
center_col = floor(cols/2);

% Define first reference color to be colr
ref_colors(1,:) = [L(center_row,center_col) a(center_row,center_col) b(center_row,center_col)];

flag = 0;
i = 1;
j = 1;
while(i <= rows)        % perform initial segmentation
    while(i <= rows && flag == 0)
        while(j <= cols && flag == 0)
            k = 1;
            min_dist = 1000;
            index = 1;
            while(k <= num_colors)
                dist = sqrt(x*(ref_colors(k,1) - L(i,j))^2 + y*(ref_colors(k,2) - a(i,j))^2 + z*(ref_colors(k,3) - b(i,j))^2);
                if(min_dist > dist)
                    min_dist = double(dist);
                    index = k;
                end
                k = k + 1;
            end
            if(j == 117)
                cow = 1;
            end
            if(min_dist > Dist_Threshold && num_colors < max_num_colors)
                ref_colors(num_colors+1,:) = [L(i,j) a(i,j) b(i,j)];
                num_colors = num_colors + 1;
                flag = 1;
                i = 0;
                j = 0;
            else
                LabelMatrix(i,j) = index;
            end
            j = j + 1;
        end
        j = 1;
        i = i + 1;
    end
    flag = 0;
end

% Go through image once more to get more accurate values for the different regions
ref_color_L_avg = zeros(50,1);
ref_color_a_avg = zeros(50,1);
ref_color_b_avg = zeros(50,1);
color_count = zeros(50,1);
for i = 1:rows
    for j = 1:cols
        index = LabelMatrix(i,j);
        ref_color_L_avg(index) = ref_color_L_avg(index) + L(i,j);
        ref_color_a_avg(index) = ref_color_a_avg(index) + a(i,j);
        ref_color_b_avg(index) = ref_color_b_avg(index) + b(i,j);
        color_count(index) = color_count(index) + 1;
    end
end
ref_color_L_avg = ref_color_L_avg ./ color_count;
ref_color_a_avg = ref_color_a_avg ./ color_count;
ref_color_b_avg = ref_color_b_avg ./ color_count;

for i = 1:num_colors
    ref_colors(i,1) = ref_color_L_avg(i);
    ref_colors(i,2) = ref_color_a_avg(i);
    ref_colors(i,3) = ref_color_b_avg(i);
end

return

== matlab function Blob_Analysis/Segmented Image/Display Image ==
  data: LabelMatrix input double; ref_colors input double; L output double; a output double; b output double
function [L, a, b] = Display_Image(LabelMatrix, ref_colors)


% Initialize
[rows,cols] = size(LabelMatrix);
L = zeros(rows,cols);
a = zeros(rows,cols);
b = zeros(rows,cols);


% Allow only colors in specified range
for r = 1:rows
    for c = 1:cols
        
        L(r,c) = ref_colors(LabelMatrix(r,c), 1);
        a(r,c) = ref_colors(LabelMatrix(r,c), 2);
        b(r,c) = ref_colors(LabelMatrix(r,c), 3);
        
    end
end


return

== matlab function make_color_range ==
  data: a_range output double; b_range output double; white_al input double; white_au input double; white_bl input double; white_bu input double; black_al input double; black_au input double; black_bl input double; black_bu input double; blue_al input double; blue_au input double; blue_bl input double; blue_bu input double; red_al input double; red_au input double; red_bl input double; red_bu input double; orange_al input double; orange_au input double; orange_bl input double; orange_bu input double; yellow_al input double; yellow_au input double; yellow_bl input double; yellow_bu input double; green_al input double; green_au input double; green_bl input double; green_bu input double
function [a_range, b_range] = make_color_range(white_al, white_au, white_bl, white_bu, black_al, black_au, black_bl, black_bu, blue_al, blue_au, blue_bl, blue_bu, red_al, red_au, red_bl, red_bu, orange_al, orange_au, orange_bl, orange_bu, yellow_al, yellow_au, yellow_bl, yellow_bu, green_al, green_au, green_bl, green_bu)

% This function forms two compact matrices which pass all color range
%   information to other functions in the model


% Initialize
a_range = zeros(2, 7);
b_range = zeros(2, 7);


% Assign values to color range matrices
a_range(1, 1) = white_al;
a_range(2, 1) = white_au;
b_range(1, 1) = white_bl;
b_range(2, 1) = white_bu;

a_range(1, 2) = black_al;
a_range(2, 2) = black_au;
b_range(1, 2) = black_bl;
b_range(2, 2) = black_bu;

a_range(1, 3) = blue_al;
a_range(2, 3) = blue_au;
b_range(1, 3) = blue_bl;
b_range(2, 3) = blue_bu;

a_range(1, 4) = red_al;
a_range(2, 4) = red_au;
b_range(1, 4) = red_bl;
b_range(2, 4) = red_bu;

a_range(1, 5) = orange_al;
a_range(2, 5) = orange_au;
b_range(1, 5) = orange_bl;
b_range(2, 5) = orange_bu;

a_range(1, 6) = yellow_al;
a_range(2, 6) = yellow_au;
b_range(1, 6) = yellow_bl;
b_range(2, 6) = yellow_bu;

a_range(1, 7) = green_al;
a_range(2, 7) = green_au;
b_range(1, 7) = green_bl;
b_range(2, 7) = green_bu;


return
